simulink model "testall"  (R2016b)
settings: Solver=VariableStepAuto  StartTime=0.0  StopTime=10.0  FixedStep=1e-7  MinStep=1e-8  RelTol=1e-3
undefined symbols (not defined in the file): fd_d, fd_i, fd_p, Kii, Kpi, me, mj2, mj3, plan, pmsm, q_init, tb, ts, X, Y, Z
libraries: nesl_utility x26, sm_lib x18, fl_lib x11, simulink x8, pe_lib x4, sdl_lib x1, pePwmGeneratorTwoLevel x1
(part 2 of 2)

== matlab function testall/gen-torque ==
  data: q input; t1 output; dq input; ddq input; t2 output; t3 output; pmsm parameter
function [t1,t2,t3] = fcn(q, dq, ddq, pmsm)

g = 9.8;
m1 = 10;
m2 = 17.4;
m3 = 4.8;

Iz1 = 0.35;
Ix2 = 0.13;
Iy2 = 0.524;
Iz2 = 0.539;
Ix3 = 0.066;
Iy3 = 0.0125;
Iz3 = 0.086;

p12 = -0.198;
p2c = 0.025;
p3c = 0.05;
p23x = 0.4318;
p23y = -0.0203;
p23z = -0.0453;

q1 = q(1); dq1 = dq(1); ddq1 = ddq(1);
q2 = q(2); dq2 = dq(2); ddq2 = ddq(2);
q3 = q(3); dq3 = dq(3); ddq3 = ddq(3);

t1 = (Ix2*ddq1)/2 + (Ix3*ddq1)/2 + (Iy2*ddq1)/2 + (Iy3*ddq1)/2 + Iz1*ddq1 + ddq1*m2*p12^2 + ddq1*m3*p12^2 + (ddq1*m3*p23x^2)/2 + (ddq1*m3*p23y^2)/2 + ddq1*m3*p23z^2 + ddq1*m2*p2c^2 + (ddq1*m3*p3c^2)/2 - (Ix2*ddq1*cos(2*q2))/2 + (Iy2*ddq1*cos(2*q2))/2 + (Ix3*ddq1*cos(2*q2 + 2*q3))/2 - (Iy3*ddq1*cos(2*q2 + 2*q3))/2 - 2*ddq1*m3*p12*p23z - 2*ddq1*m2*p12*p2c + (ddq1*m3*p23x^2*cos(2*q2))/2 - (ddq1*m3*p23y^2*cos(2*q2))/2 - (ddq1*m3*p3c^2*cos(2*q2 + 2*q3))/2 + Ix2*dq1*dq2*sin(2*q2) - Iy2*dq1*dq2*sin(2*q2) - Ix3*dq1*dq2*sin(2*q2 + 2*q3) - Ix3*dq1*dq3*sin(2*q2 + 2*q3) + Iy3*dq1*dq2*sin(2*q2 + 2*q3) + Iy3*dq1*dq3*sin(2*q2 + 2*q3) - ddq1*m3*p23y*p3c*cos(2*q2 + q3) - ddq1*m3*p23x*p3c*sin(2*q2 + q3) - dq2^2*m3*p12*p3c*sin(q2 + q3) - dq3^2*m3*p12*p3c*sin(q2 + q3) + dq2^2*m3*p23z*p3c*sin(q2 + q3) + dq3^2*m3*p23z*p3c*sin(q2 + q3) + dq2^2*m3*p12*p23x*cos(q2) - dq2^2*m3*p23x*p23z*cos(q2) - ddq1*m3*p23x*p23y*sin(2*q2) - dq2^2*m3*p12*p23y*sin(q2) + dq2^2*m3*p23y*p23z*sin(q2) - dq1*dq2*m3*p23x^2*sin(2*q2) + dq1*dq2*m3*p23y^2*sin(2*q2) + ddq2*m3*p12*p3c*cos(q2 + q3) + ddq3*m3*p12*p3c*cos(q2 + q3) - ddq2*m3*p23z*p3c*cos(q2 + q3) - ddq3*m3*p23z*p3c*cos(q2 + q3) + dq1*dq2*m3*p3c^2*sin(2*q2 + 2*q3) + dq1*dq3*m3*p3c^2*sin(2*q2 + 2*q3) + ddq2*m3*p12*p23y*cos(q2) - ddq2*m3*p23y*p23z*cos(q2) + ddq1*m3*p23y*p3c*cos(q3) + ddq2*m3*p12*p23x*sin(q2) - ddq2*m3*p23x*p23z*sin(q2) - ddq1*m3*p23x*p3c*sin(q3) - 2*dq2*dq3*m3*p12*p3c*sin(q2 + q3) + 2*dq2*dq3*m3*p23z*p3c*sin(q2 + q3) - dq1*dq3*m3*p23x*p3c*cos(q3) - dq1*dq3*m3*p23y*p3c*sin(q3) - 2*dq1*dq2*m3*p23x*p3c*cos(2*q2 + q3) - dq1*dq3*m3*p23x*p3c*cos(2*q2 + q3) + 2*dq1*dq2*m3*p23y*p3c*sin(2*q2 + q3) + dq1*dq3*m3*p23y*p3c*sin(2*q2 + q3) - 2*dq1*dq2*m3*p23x*p23y*cos(2*q2);
t2 = Iz2*ddq2 + Iz3*ddq2 + Iz3*ddq3 + ddq2*m3*p23x^2 + ddq2*m3*p23y^2 + ddq2*m3*p3c^2 + ddq3*m3*p3c^2 - (Ix2*dq1^2*sin(2*q2))/2 + (Iy2*dq1^2*sin(2*q2))/2 + (Ix3*dq1^2*sin(2*q2 + 2*q3))/2 - (Iy3*dq1^2*sin(2*q2 + 2*q3))/2 - g*m3*p3c*sin(q2 + q3) + g*m3*p23x*cos(q2) - g*m3*p23y*sin(q2) + (dq1^2*m3*p23x^2*sin(2*q2))/2 - (dq1^2*m3*p23y^2*sin(2*q2))/2 - (dq1^2*m3*p3c^2*sin(2*q2 + 2*q3))/2 - dq3^2*m3*p23x*p3c*cos(q3) - dq3^2*m3*p23y*p3c*sin(q3) + dq1^2*m3*p23x*p3c*cos(2*q2 + q3) - dq1^2*m3*p23y*p3c*sin(2*q2 + q3) + dq1^2*m3*p23x*p23y*cos(2*q2) + ddq1*m3*p12*p3c*cos(q2 + q3) - ddq1*m3*p23z*p3c*cos(q2 + q3) + ddq1*m3*p12*p23y*cos(q2) - ddq1*m3*p23y*p23z*cos(q2) + 2*ddq2*m3*p23y*p3c*cos(q3) + ddq3*m3*p23y*p3c*cos(q3) + ddq1*m3*p12*p23x*sin(q2) - ddq1*m3*p23x*p23z*sin(q2) - 2*ddq2*m3*p23x*p3c*sin(q3) - ddq3*m3*p23x*p3c*sin(q3) - 2*dq2*dq3*m3*p23x*p3c*cos(q3) - 2*dq2*dq3*m3*p23y*p3c*sin(q3);
t3 = Iz3*ddq2 + Iz3*ddq3 + ddq2*m3*p3c^2 + ddq3*m3*p3c^2 + (Ix3*dq1^2*sin(2*q2 + 2*q3))/2 - (Iy3*dq1^2*sin(2*q2 + 2*q3))/2 - g*m3*p3c*sin(q2 + q3) - (dq1^2*m3*p3c^2*sin(2*q2 + 2*q3))/2 + (dq1^2*m3*p23x*p3c*cos(q3))/2 + dq2^2*m3*p23x*p3c*cos(q3) + (dq1^2*m3*p23y*p3c*sin(q3))/2 + dq2^2*m3*p23y*p3c*sin(q3) + (dq1^2*m3*p23x*p3c*cos(2*q2 + q3))/2 - (dq1^2*m3*p23y*p3c*sin(2*q2 + q3))/2 + ddq1*m3*p12*p3c*cos(q2 + q3) - ddq1*m3*p23z*p3c*cos(q2 + q3) + ddq2*m3*p23y*p3c*cos(q3) - ddq2*m3*p23x*p3c*sin(q3);

t3 = t3 + pmsm.J * pmsm.gear^2 * ddq3;

end

== matlab function testall/gen-trajectory ==
  data: u input; q output; dq output; ddq output; tf parameter double; tb parameter; q_init parameter; plan parameter
function [q,dq,ddq] = fcn(u, tf, tb, q_init, plan)
% goto the starting point
if u < tf
    q = 3*q_init/tf^2*u^2 -2*q_init/tf^3*u^3;
    dq = 6*q_init/tf^2*u - 6*q_init/tf^3*u^2;
    ddq = 6*q_init/tf^2 - 12*q_init/tf^3*u;
else if u < tb
    q = q_init;
    dq = zeros(3,1);
    ddq = zeros(3,1);
else
    % start to draw a circle
    tt = 1e-3;
    t = u - tb;
    id = round(t/tt);
    if id == 0
        id = 1;
    end
    if id <= size(plan.q, 2)
        q = plan.q(:,id);
        dq = plan.dq(:,id);
        ddq = plan.ddq(:,id);
    else
        q = plan.q(:,end);
        dq = zeros(3,1);
        ddq = zeros(3,1);
    end
    end

end

== matlab function testall/PMSM Acutator3/MATLAB Function ==
  data: ud input; u data_store_memory
function fcn(ud)
global u;
if ud < 8
    u = 10;
else
    if ud > 0.9 * u
        u = u/0.9;
    else if ud < 0.7 * u
        u = u*0.7;
        end
    end

end

== matlab function testall/gen-TL ==
  data: q input; dq input; t3 output
function t3  = fcn(q,dq)
    
g = 9.8;
m3 = 4.8;

Ix3 = 0.066;
Iy3 = 0.0125;

p12 = -0.198;
p2c = 0.025;
p3c = 0.05;
p23x = 0.4318;
p23y = -0.0203;
p23z = -0.0453;

q1 = q(1); dq1 = dq(1); 
q2 = q(2); dq2 = dq(2);
q3 = q(3); dq3 = dq(3); 

mp = m3*p3c;
mp2 = m3*p3c^2;

G3 = - mp*sin(q2 + q3)*g;
V3 = dq1^2 * ( (Ix3 - Iy3 - mp2)*sin(2*q2 + 2*q3)/2 + ...
    mp*(p23x*cos(q3)/2 + p23y*sin(q3)/2) + ...
	mp*(p23x*cos(2*q2 + q3)/2 - p23y*sin(2*q2 + q3)/2) ) + ...
 dq2^2 * ( mp*(p23x*cos(q3) + p23y*sin(q3)) );

t3 = V3 + G3;

end

== matlab function testall/gen-J ==
  data: q input; j1 output; j2 output; j3 output; pmsm parameter
function [j1,j2,j3] = fcn(q, pmsm)

g = 9.8;
m3 = 4.8;

p3c = 0.05;
p23x = 0.4318;
p23y = -0.0203;

q1 = q(1); 
q2 = q(2);
q3 = q(3);

j1 = pmsm.J * pmsm.gear^2;
j2 = j1 - g*m3*p3c*sin(q2 + q3) + g*m3*p23x*cos(q2) - g*m3*p23y*sin(q2);
j3 = j1 - m3*p3c*sin(q2 + q3)*g;

end
